simulink model "Tecs"  (R2023b)
settings: Solver=ode4  StartTime=0.0  StopTime=50  FixedStep=.02  RelTol=1e-3
values from neighbouring files (symbols this model uses):
  gravity = Airplane_data(52)    [Data_edit.m]
libraries: simulink x11
settings Model: Creator=Saif Mohamed  LastModifiedBy=saifg

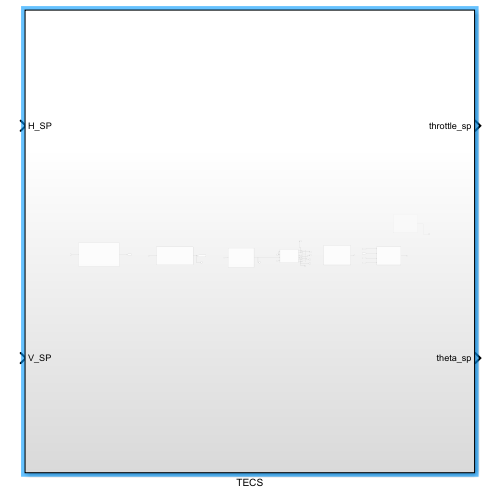
[thumbnail: Simulink's stored preview of the top-level diagram]
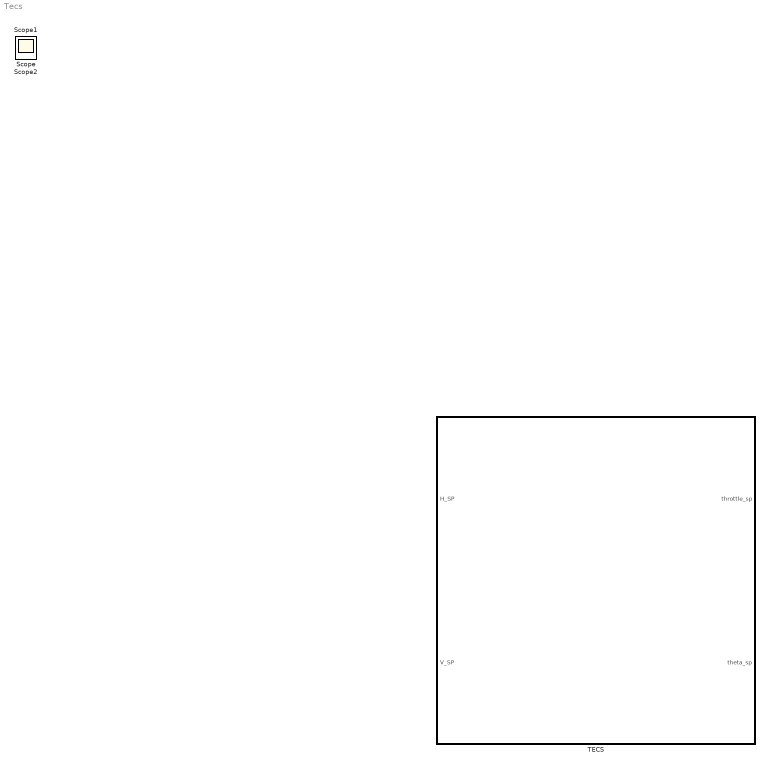
== system Tecs ==
  TECS : Subsystem
  Scope : Scope
  Scope1 : Scope
  Scope2 : Scope

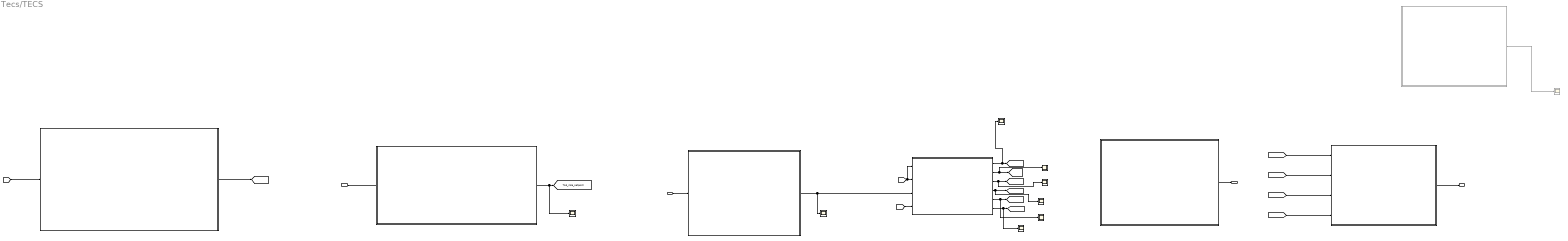
== system Tecs/TECS ==
  H_SP : Inport
  V_SP : Inport  Port=2
  Scope{,1..7} (8 alike) : Scope
  Scope9 : Scope  Commented=on
  _update_pitch_setpoint : Subsystem
  runAltitudeControllerSmoothVelocity : Subsystem
  update_energy_estimates : Subsystem
  update_pitch_setpoint : Subsystem  Commented=on
  update_speed_setpoint : Subsystem
  update_speed_states : Subsystem
  update_throttle_setpoint : Subsystem
  throttle_sp : Outport
  theta_sp : Outport  Port=2
  tag scope: SEB_error=global, SKE_rate=global, SKE_rate_setpoint=global, SPE_rate=global, SPE_rate_setpoint=global, STE_error=global, TAS_rate_setpoint=global, tas_state_output=global
  wires:
  update_speed_setpoint/1(TAS_rate_setpoint) -> Scope/1, [TAS_rate_setpoint]
  update_energy_estimates/4(SKE_rate_setpoint) -> Scope5/1, [SKE_rate_setpoint]
  update_energy_estimates/3(SPE_rate_setpoint) -> Scope4/1, [SPE_rate_setpoint]
  update_energy_estimates/5(SPE_rate) -> Scope6/1, [SPE_rate]
  update_speed_states/1(tas_state) -> [tas_state_output]  "tas_state"
  update_energy_estimates/6(SKE_rate) -> Scope7/1, [SKE_rate]
  V_SP/1 -> update_speed_setpoint/1(TAS_setpoint)
  update_energy_estimates/1(STE_error) -> Scope2/1, [STE_error]
  update_energy_estimates/2(SEB_error) -> Scope3/1, [SEB_error]
  update_pitch_setpoint/1(_last_pitch_setpoint) -> Scope9/1
  [Z] -> update_energy_estimates/1(hgt_setpoint), update_energy_estimates/2(vert_pos_state z from (6DoF))
  [w_e] -> update_energy_estimates/4(vert_vel_state)
  H_SP/1 -> runAltitudeControllerSmoothVelocity/1(H_Desired)
  runAltitudeControllerSmoothVelocity/1(hgt_rate_setpoint) -> Scope1/1, update_energy_estimates/3(hgt_rate_setpoint)
  update_throttle_setpoint/1(last_throttle_setpoint) -> throttle_sp/1
  [SPE_rate] -> _update_pitch_setpoint/2(SPE_Rate)
  _update_pitch_setpoint/1(_last_pitch_setpoint) -> theta_sp/1
  [SKE_rate] -> _update_pitch_setpoint/3(SKE_Rate)
  [SPE_rate_setpoint] -> _update_pitch_setpoint/1(SPE_rate_setpoint)
  [SKE_rate_setpoint] -> _update_pitch_setpoint/4(SKE_rate_setpoint)
  [V_tot] -> update_speed_states/1(EAS)

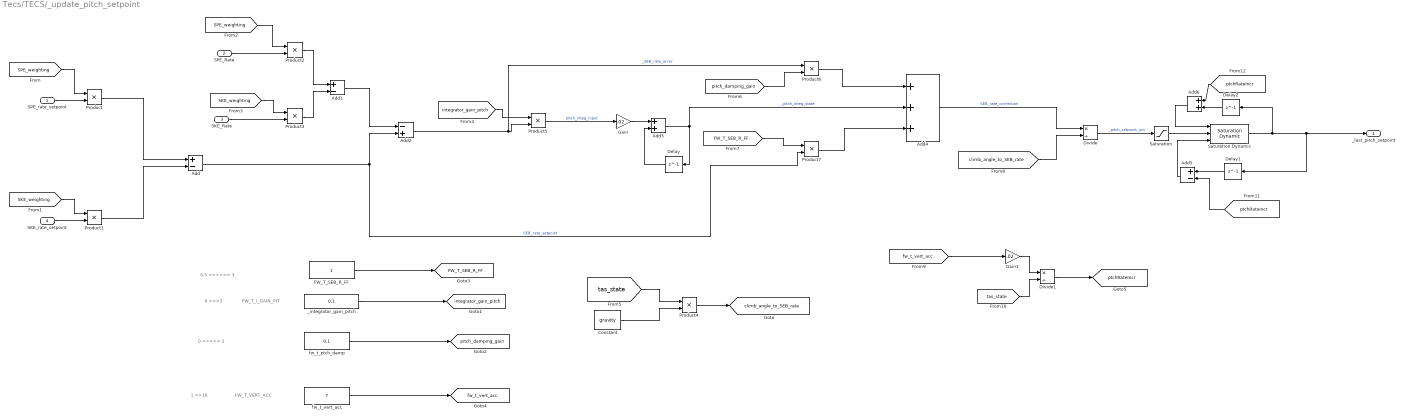
== system Tecs/TECS/_update_pitch_setpoint ==
  note: 0 >>>>> 2
  note: 0.5 >>>>>> 3
  note: FW_T_VERT_ACC
  note: 1 >>10
  note: 0 >>>2
  note: FW_T_I_GAIN_PIT
  SPE_rate_setpoint : Inport
  SPE_Rate : Inport  Port=2
  SKE_Rate : Inport  Port=3
  SKE_rate_setpoint : Inport  Port=4
  Add : Sum  Inputs=+-
  Add1 : Sum  Inputs=+-
  Add2 : Sum  Inputs=-+
  Add3 : Sum
  Add4 : Sum  Inputs=+++
  Add5 : Sum  Inputs=+-
  Add6 : Sum
  Constant : Constant  Value=gravity
  Delay : Delay  DelayLength=1
  Delay1 : Delay  DelayLength=1
  Delay2 : Delay  DelayLength=1
  Divide : Product  Inputs=*/
  Divide1 : Product  Inputs=*/
  FW_T_SEB_R_FF : Constant
  Gain : Gain  Gain=.02
  Gain1 : Gain  Gain=.02
  Product{,1..7} (8 alike) : Product
  Saturation : Saturate
  Saturation Dynamic : simulink/Discontinuities/Saturation Dynamic  OutMin=[]  OutMax=[]  OutDataTypeStr=Inherit: Same as second input  OutDataType=fixdt(1, 16)  OutScaling=2^-10  DoSatur=off
  _integrator_gain_pitch : Constant  Value=0.1
  fw_t_ptch_damp : Constant  Value=0.1
  fw_t_vert_acc : Constant  Value=7
  _last_pitch_setpoint : Outport
  tag scope: FW_T_SEB_R_FF=global, climb_angle_to_SEB_rate=global, fw_t_vert_acc=global, integrator_gain_pitch=global, pitch_damping_gain=global, ptchRateIncr=global
  wires:
  SKE_rate_setpoint/1 -> Product1/2
  SPE_rate_setpoint/1 -> Product/2
  Product/1 -> Add/1
  Product1/1 -> Add/2
  [SPE_weighting] -> Product/1
  [SKE_weighting] -> Product1/1
  SPE_Rate/1 -> Product2/2
  [SPE_weighting] -> Product2/1
  SKE_Rate/1 -> Product3/2
  [SKE_weighting] -> Product3/1
  Product3/1 -> Add1/2
  Product2/1 -> Add1/1
  Add/1 -> Product7/2, Add2/2  "SEB_rate_setpoint"
  Add1/1 -> Add2/1
  Add2/1 -> Product6/1, Product5/2  "_SEB_rate_error"
  [tas_state] -> Product4/1
  Constant/1 -> Product4/2
  Product4/1 -> [climb_angle_to_SEB_rate]
  _integrator_gain_pitch/1 -> [integrator_gain_pitch]
  [integrator_gain_pitch] -> Product5/1
  Product5/1 -> Gain/1  "pitch_integ_input"
  Gain/1 -> Add3/1
  Add3/1 -> Add4/2, Delay/1  "_pitch_integ_state"
  Delay/1 -> Add3/2
  fw_t_ptch_damp/1 -> [pitch_damping_gain]
  [pitch_damping_gain] -> Product6/2
  Product6/1 -> Add4/1
  FW_T_SEB_R_FF/1 -> [FW_T_SEB_R_FF]
  [FW_T_SEB_R_FF] -> Product7/1
  Product7/1 -> Add4/3
  Add4/1 -> Divide/1  "SEB_rate_correction"
  [climb_angle_to_SEB_rate] -> Divide/2
  Divide/1 -> Saturation/1  "_pitch_setpoint_unc"
  fw_t_vert_acc/1 -> [fw_t_vert_acc]
  [tas_state] -> Divide1/2
  [fw_t_vert_acc] -> Gain1/1
  Gain1/1 -> Divide1/1
  Divide1/1 -> [ptchRateIncr]
  Saturation/1 -> Saturation Dynamic/2
  Saturation Dynamic/1 -> Delay2/1, _last_pitch_setpoint/1, Delay1/1
  Delay1/1 -> Add5/1
  [ptchRateIncr] -> Add5/2
  Add5/1 -> Saturation Dynamic/3
  Delay2/1 -> Add6/2
  [ptchRateIncr] -> Add6/1
  Add6/1 -> Saturation Dynamic/1

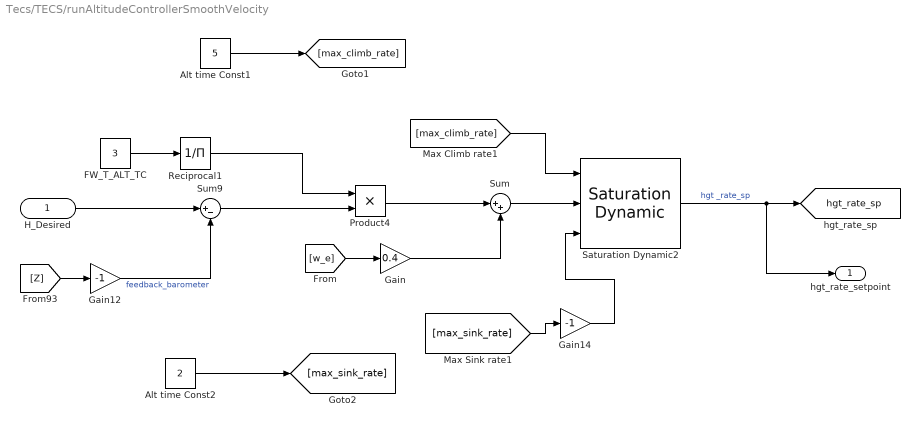
== system Tecs/TECS/runAltitudeControllerSmoothVelocity ==
  H_Desired : Inport
  Alt time Const1 : Constant  Value=5
  Alt time Const2 : Constant  Value=2
  FW_T_ALT_TC : Constant  Value=3
  Gain : Gain  Gain=0.4
  Gain12 : Gain  Gain=-1
  Gain14 : Gain  Gain=-1
  Product4 : Product
  Reciprocal1 : Product  Inputs=/
  Saturation Dynamic2 : simulink/Discontinuities/Saturation Dynamic  OutMin=[]  OutMax=[]  OutDataTypeStr=Inherit: Same as second input  OutDataType=fixdt(1, 16)  OutScaling=2^-10  DoSatur=off
  Sum : Sum  Inputs=|++
  Sum9 : Sum  Inputs=|+-
  hgt_rate_setpoint : Outport
  tag scope: hgt_rate_sp=global
  wires:
  Gain12/1 -> Sum9/2  "feedback_barometer"
  FW_T_ALT_TC/1 -> Reciprocal1/1
  H_Desired/1 -> Sum9/1
  [Z] -> Gain12/1
  Sum9/1 -> Product4/2
  [max_sink_rate] -> Gain14/1
  Reciprocal1/1 -> Product4/1
  Gain14/1 -> Saturation Dynamic2/3
  Saturation Dynamic2/1 -> hgt_rate_setpoint/1, [hgt_rate_sp]  "hgt _rate_sp"
  [max_climb_rate] -> Saturation Dynamic2/1
  Alt time Const1/1 -> [max_climb_rate]
  Alt time Const2/1 -> [max_sink_rate]
  [w_e] -> Gain/1
  Sum/1 -> Saturation Dynamic2/2
  Product4/1 -> Sum/1
  Gain/1 -> Sum/2

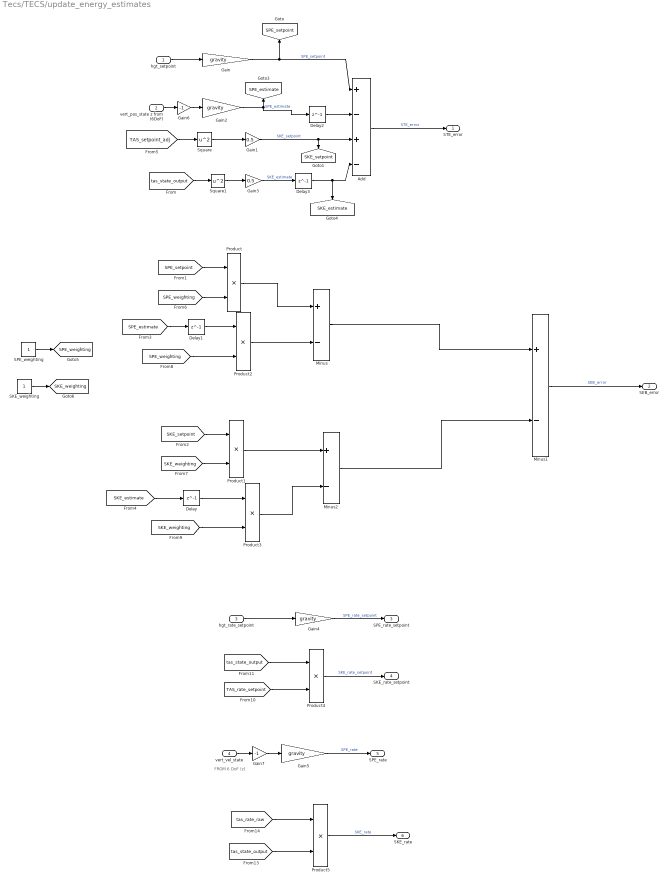
== system Tecs/TECS/update_energy_estimates ==
  note: FROM 6 DoF (z)
  hgt_setpoint : Inport
  vert_pos_state z from (6DoF) : Inport  Port=2
  hgt_rate_setpoint : Inport  Port=3
  vert_vel_state : Inport  Port=4
  Add : Sum  Inputs=+-+-
  Delay{,1..3} (4 alike) : Delay  DelayLength=1
  Gain{,2,4..5} (4 alike) : Gain  Gain=gravity
  Gain1 : Gain  Gain=0.5
  Gain3 : Gain  Gain=0.5
  Gain6 : Gain  Gain=-1
  Gain7 : Gain  Gain=-1
  Minus : Sum  Inputs=+-
  Minus1 : Sum  Inputs=+-
  Minus2 : Sum  Inputs=+-
  Product{,1..5} (6 alike) : Product
  SKE_weighting : Constant
  SPE_weighting : Constant
  Square : Math  Operator=square
  Square1 : Math  Operator=square
  STE_error : Outport
  SEB_error : Outport  Port=2
  SPE_rate_setpoint : Outport  Port=3
  SKE_rate_setpoint : Outport  Port=4
  SPE_rate : Outport  Port=5
  SKE_rate : Outport  Port=6
  tag scope: SKE_estimate=global, SKE_setpoint=global, SKE_weighting=global, SPE_estimate=global, SPE_setpoint=global, SPE_weighting=global
  wires:
  [SPE_weighting] -> Product2/2
  SKE_weighting/1 -> [SKE_weighting]
  [SKE_weighting] -> Product1/2
  vert_pos_state z from (6DoF)/1 -> Gain6/1
  [SKE_estimate] -> Delay/1
  [tas_rate_raw] -> Product5/1
  Square1/1 -> Gain3/1
  [SKE_setpoint] -> Product1/1
  [SPE_weighting] -> Product/2
  Product5/1 -> SKE_rate/1  "SKE_rate"
  [SKE_weighting] -> Product3/2
  [tas_state_output] -> Product4/1
  Gain3/1 -> Delay3/1  "SKE_estimate"
  hgt_setpoint/1 -> Gain/1
  Gain2/1 -> Delay2/1, [SPE_estimate]  "SPE_estimate"
  [tas_state_output] -> Square1/1
  [SPE_estimate] -> Delay1/1
  vert_vel_state/1 -> Gain7/1
  Minus/1 -> Minus1/1
  [tas_state_output] -> Product5/2
  Gain/1 -> Add/1, [SPE_setpoint]  "SPE_setpoint"
  Minus2/1 -> Minus1/2
  Gain1/1 -> [SKE_setpoint], Add/3  "SKE_setpoint"
  Product3/1 -> Minus2/2
  [TAS_setpoint_adj] -> Square/1
  Square/1 -> Gain1/1
  [SPE_setpoint] -> Product/1
  Product/1 -> Minus/1
  Add/1 -> STE_error/1  "STE_error"
  hgt_rate_setpoint/1 -> Gain4/1
  [TAS_rate_setpoint] -> Product4/2
  Gain5/1 -> SPE_rate/1  "SPE_rate"
  SPE_weighting/1 -> [SPE_weighting]
  Minus1/1 -> SEB_error/1  "SEB_error"
  Product4/1 -> SKE_rate_setpoint/1  "SKE_rate_setpoint"
  Gain4/1 -> SPE_rate_setpoint/1  "SPE_rate_setpoint"
  Delay/1 -> Product3/1
  Delay1/1 -> Product2/1
  Product2/1 -> Minus/2
  Product1/1 -> Minus2/1
  Gain6/1 -> Gain2/1
  Delay2/1 -> Add/2
  Delay3/1 -> Add/4, [SKE_estimate]
  Gain7/1 -> Gain5/1

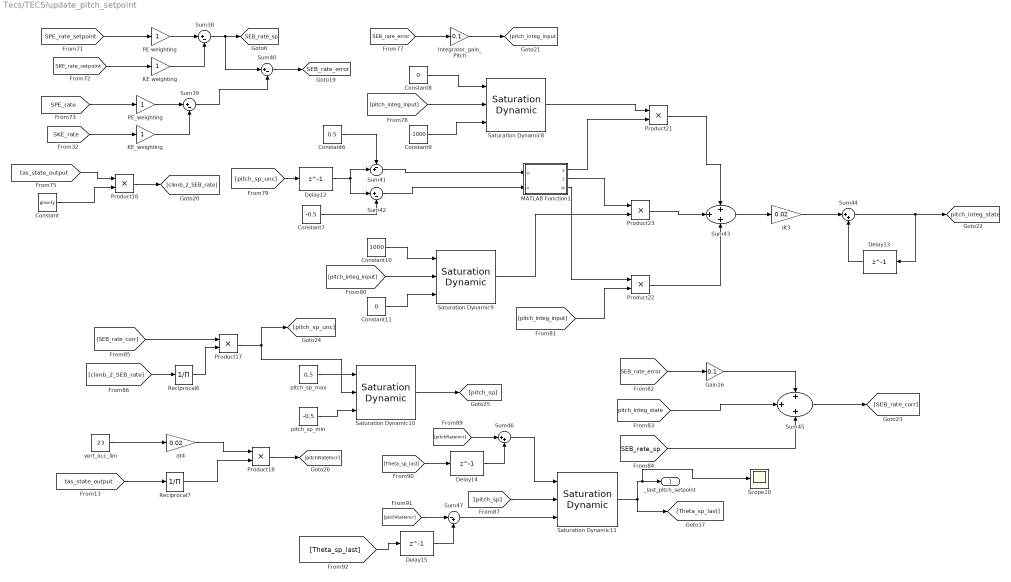
== system Tecs/TECS/update_pitch_setpoint ==
  Constant : Constant  Value=gravity
  Constant10 : Constant  Value=1000
  Constant11 : Constant  Value=0
  Constant6 : Constant  Value=0.5
  Constant7 : Constant  Value=-0.5
  Constant8 : Constant  Value=0
  Constant9 : Constant  Value=-1000
  Delay{12..15} (4 alike) : Delay  DelayLength=1  InitialCondition=0  UseCircularBuffer=on  SampleTime=0.02
  Gain16 : Gain  Gain=0.1
  Integrator_gain_Pitch : Gain  Gain=0.1
  KE weighting : Gain
  KE_weighting : Gain
  MATLAB Function1 : MATLAB Function  TreatAsAtomicUnit=on
  PE weighting : Gain
  PE_weighting : Gain
  Product{16..18,21..23} (6 alike) : Product
  Reciprocal6 : Product  Inputs=/
  Reciprocal7 : Product  Inputs=/
  Saturation Dynamic{8..11} (4 alike) : simulink/Discontinuities/Saturation Dynamic  OutMin=[]  OutMax=[]  OutDataTypeStr=Inherit: Same as second input  OutDataType=fixdt(1, 16)  OutScaling=2^-10  DoSatur=off
  Scope10 : Scope
  Sum{38..40,42} (4 alike) : Sum  Inputs=|+-
  Sum41 : Sum  Inputs=-+|
  Sum43 : Sum  Inputs=+++
  Sum44 : Sum  Inputs=|++
  Sum45 : Sum  Inputs=+++
  Sum46 : Sum  Inputs=|++
  Sum47 : Sum  Inputs=|-+
  dt3 : Gain  Gain=0.02
  dt4 : Gain  Gain=0.02
  pitch_sp_max : Constant  Value=0.5
  pitch_sp_min : Constant  Value=-0.5
  vert_acc_lim : Constant  Value=23
  _last_pitch_setpoint : Outport
  tag scope: SEB_rate_error=global, SEB_rate_sp=global, pitch_integ_state=global
  wires:
  Product18/1 -> [pitchRateIncr]
  Saturation Dynamic9/1 -> Product23/2
  [tas_state_output] -> Reciprocal7/1
  pitch_sp_min/1 -> Saturation Dynamic10/3
  [climb_2_SEB_rate] -> Reciprocal6/1
  KE weighting/1 -> Sum38/2
  Gain16/1 -> Sum45/1
  [SEB_rate_corr] -> Product17/1
  Reciprocal7/1 -> Product18/2
  pitch_sp_max/1 -> Saturation Dynamic10/1
  [pitch_integ_input] -> Product22/2
  [SPE_rate_setpoint] -> PE weighting/1
  PE weighting/1 -> Sum38/1
  Product16/1 -> [climb_2_SEB_rate]
  Reciprocal6/1 -> Product17/2
  Delay15/1 -> Sum47/2
  [pitchRateIncr] -> Sum47/1
  Sum46/1 -> Saturation Dynamic11/1
  Delay12/1 -> Sum42/1, Sum41/2
  Delay13/1 -> Sum44/2
  [SEB_rate_sp] -> Sum45/3
  [tas_state_output] -> Product16/1
  [SEB_rate_error] -> Gain16/1
  KE_weighting/1 -> Sum39/2
  MATLAB Function1/2(z) -> Product23/1
  [pitch_integ_input] -> Saturation Dynamic9/2
  [Theta_sp_last] -> Delay15/1
  Sum45/1 -> [SEB_rate_corr]
  Product23/1 -> Sum43/2
  Constant8/1 -> Saturation Dynamic8/1
  Sum43/1 -> dt3/1
  [SKE_rate_setpoint] -> KE weighting/1
  MATLAB Function1/3(w) -> Product22/1
  Sum40/1 -> [SEB_rate_error]
  vert_acc_lim/1 -> dt4/1
  Sum39/1 -> Sum40/2
  MATLAB Function1/1(y) -> Product21/2
  Constant10/1 -> Saturation Dynamic9/1
  [pitch_sp_unc] -> Delay12/1
  Saturation Dynamic11/1 -> _last_pitch_setpoint/1, Scope10/1, [Theta_sp_last]
  Constant11/1 -> Saturation Dynamic9/3
  dt3/1 -> Sum44/1
  [pitchRateIncr] -> Sum46/1
  Product22/1 -> Sum43/3
  [pitch_integ_state] -> Sum45/2
  Integrator_gain_Pitch/1 -> [pitch_integ_input]
  Constant6/1 -> Sum41/1
  Delay14/1 -> Sum46/2
  Saturation Dynamic8/1 -> Product21/1
  Constant9/1 -> Saturation Dynamic8/3
  Constant/1 -> Product16/2
  Product21/1 -> Sum43/1
  Sum44/1 -> Delay13/1, [pitch_integ_state]
  Sum42/1 -> MATLAB Function1/2(v)
  [SEB_rate_error] -> Integrator_gain_Pitch/1
  Product17/1 -> Saturation Dynamic10/2, [pitch_sp_unc]
  PE_weighting/1 -> Sum39/1
  Sum41/1 -> MATLAB Function1/1(u)
  [pitch_integ_input] -> Saturation Dynamic8/2
  Sum47/1 -> Saturation Dynamic11/3
  [pitch_sp] -> Saturation Dynamic11/2
  Sum38/1 -> Sum40/1, [SEB_rate_sp]
  Constant7/1 -> Sum42/2
  [SPE_rate] -> PE_weighting/1
  [SKE_rate] -> KE_weighting/1
  Saturation Dynamic10/1 -> [pitch_sp]
  dt4/1 -> Product18/1
  [Theta_sp_last] -> Delay14/1

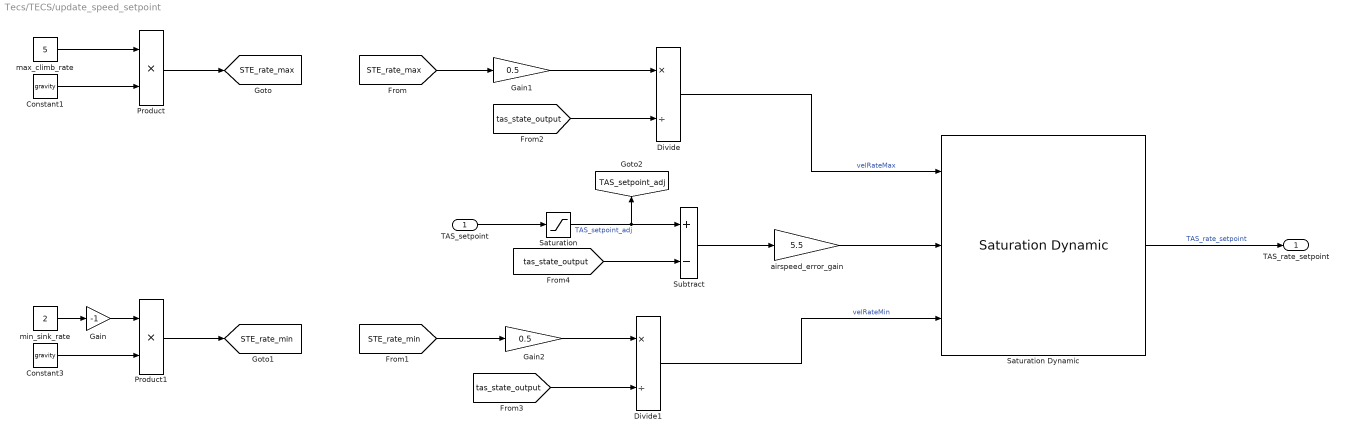
== system Tecs/TECS/update_speed_setpoint ==
  TAS_setpoint : Inport
  Constant1 : Constant  Value=gravity
  Constant3 : Constant  Value=gravity
  Divide : Product  Inputs=*/
  Divide1 : Product  Inputs=*/
  Gain : Gain  Gain=-1
  Gain1 : Gain  Gain=0.5
  Gain2 : Gain  Gain=0.5
  Product : Product
  Product1 : Product
  Saturation : Saturate  UpperLimit=50  LowerLimit=8
  Saturation Dynamic : simulink/Discontinuities/Saturation Dynamic  OutMin=[]  OutMax=[]  OutDataTypeStr=Inherit: Same as second input  OutDataType=fixdt(1, 16)  OutScaling=2^-10  DoSatur=off
  Subtract : Sum  Inputs=+-
  airspeed_error_gain : Gain  Gain=5.5
  max_climb_rate : Constant  Value=5
  min_sink_rate : Constant  Value=2
  TAS_rate_setpoint : Outport
  tag scope: STE_rate_max=global, STE_rate_min=global, TAS_setpoint_adj=global
  wires:
  Saturation Dynamic/1 -> TAS_rate_setpoint/1  "TAS_rate_setpoint"
  Divide1/1 -> Saturation Dynamic/3  "velRateMin"
  Gain2/1 -> Divide1/1
  Product/1 -> [STE_rate_max]
  [STE_rate_min] -> Gain2/1
  [tas_state_output] -> Divide1/2
  [STE_rate_max] -> Gain1/1
  airspeed_error_gain/1 -> Saturation Dynamic/2
  Divide/1 -> Saturation Dynamic/1  "velRateMax"
  Gain1/1 -> Divide/1
  [tas_state_output] -> Subtract/2
  Constant3/1 -> Product1/2
  max_climb_rate/1 -> Product/1
  min_sink_rate/1 -> Gain/1
  Saturation/1 -> Subtract/1, [TAS_setpoint_adj]  "TAS_setpoint_adj"
  Constant1/1 -> Product/2
  [tas_state_output] -> Divide/2
  TAS_setpoint/1 -> Saturation/1
  Subtract/1 -> airspeed_error_gain/1
  Product1/1 -> [STE_rate_min]
  Gain/1 -> Product1/1

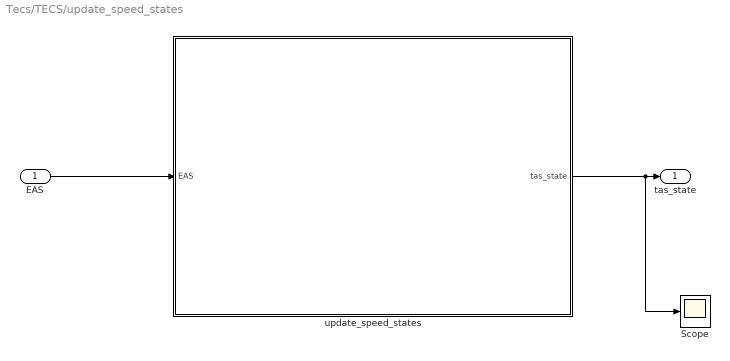
== system Tecs/TECS/update_speed_states ==
  EAS : Inport
  Scope : Scope
  update_speed_states : Subsystem
  tas_state : Outport
  wires:
  EAS/1 -> update_speed_states/1(EAS)
  update_speed_states/1(tas_state) -> Scope/1, tas_state/1

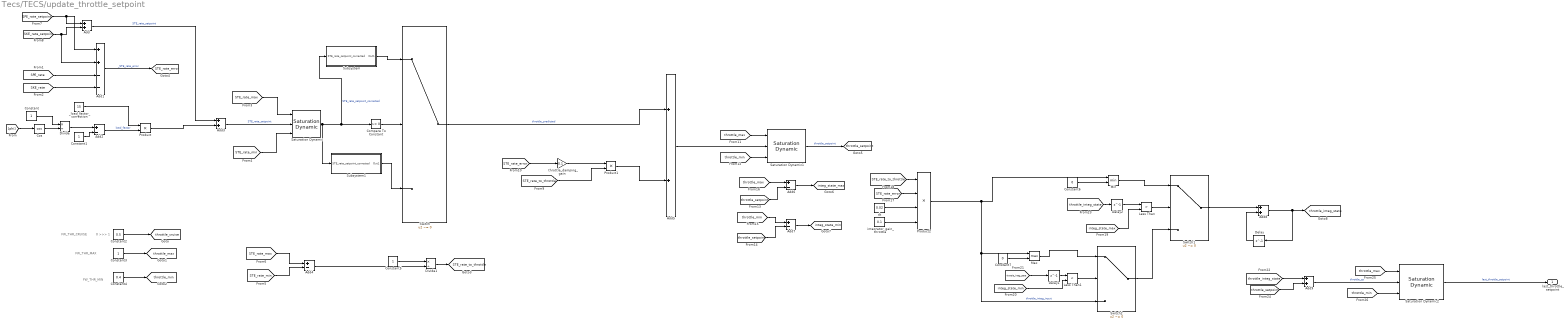
== system Tecs/TECS/update_throttle_setpoint ==
  note: FW_THR_MIN
  note: FW_THR_MAX
  note: FW_THR_CRUISE
  note: 0 >>> 1
  Add{,3,5,8..9} (5 alike) : Sum
  Add1 : Sum  Inputs=++--
  Add{2,4,6..7} (4 alike) : Sum  Inputs=+-
  Compare To Constant : simulink/Logic and Bit Operations/Compare To Constant  relop=>=  const=0  OutDataTypeStr=boolean
  Constant{,1,3,5} (4 alike) : Constant
  Constant2 : Constant  Value=0.5
  Constant4 : Constant  Value=0.4
  Constant6 : Constant  Value=0
  Constant7 : Constant  Value=0
  Cos : Trigonometry  Operator=cos
  Delay : Delay  DelayLength=1
  Delay1 : Delay  DelayLength=1
  Delay2 : Delay  DelayLength=1
  Divide : Product  Inputs=*/
  Divide1 : Product  Inputs=*/
  Less Than : RelationalOperator  Operator=>  OutDataTypeStr=boolean  RndMeth=Simplest  InputSameDT=off
  Less Than1 : RelationalOperator  Operator=<  OutDataTypeStr=boolean  RndMeth=Simplest  InputSameDT=off
  Max : MinMax  Function=max  Inputs=2
  Min : MinMax  Inputs=2
  Product : Product
  Product1 : Product
  Product2 : Product  Inputs=4
  Saturation Dynamic : simulink/Discontinuities/Saturation Dynamic  OutMin=[]  OutMax=[]  OutDataTypeStr=Inherit: Same as second input  OutDataType=fixdt(1, 16)  OutScaling=2^-10  DoSatur=off
  Saturation Dynamic1 : simulink/Discontinuities/Saturation Dynamic  OutMin=[]  OutMax=[]  OutDataTypeStr=Inherit: Same as second input  OutDataType=fixdt(1, 16)  OutScaling=2^-10  DoSatur=off
  Saturation Dynamic2 : simulink/Discontinuities/Saturation Dynamic  OutMin=[]  OutMax=[]  OutDataTypeStr=Inherit: Same as second input  OutDataType=fixdt(1, 16)  OutScaling=2^-10  DoSatur=off
  Subsystem : Subsystem
  Subsystem1 : Subsystem
  Switch : Switch  Criteria=u2 ~= 0  SaturateOnIntegerOverflow=off  InputSameDT=off
  Switch1 : Switch  Criteria=u2 ~= 0  SaturateOnIntegerOverflow=off  InputSameDT=off
  Switch2 : Switch  Criteria=u2 ~= 0  SaturateOnIntegerOverflow=off  InputSameDT=off
  _load_factor_correction : Constant  Value=15
  dt : Constant  Value=0.02
  integrator_gain_throttle : Constant  Value=0.1
  throttle_damping_gain : Gain  Gain=0.1
  last_throttle_setpoint : Outport
  tag scope: STE_rate_error=global, STE_rate_to_throttle=global, integ_state_max=global, integ_state_min=global, throttle_cruise=global, throttle_integ_state=global, throttle_max=global, throttle_min=global, throttle_setpoint=global
  wires:
  [SKE_rate_setpoint] -> Add1/2, Add/2
  [SPE_rate_setpoint] -> Add1/1, Add/1
  Add/1 -> Add3/1  "STE_rate_setpoint"
  [SPE_rate] -> Add1/3
  [SKE_rate] -> Add1/4
  Add1/1 -> [STE_rate_error]  "_STE_rate_error"
  [phi] -> Cos/1
  Cos/1 -> Divide/2
  Constant/1 -> Divide/1
  Divide/1 -> Add2/1
  Constant1/1 -> Add2/2
  Add2/1 -> Product/2  "load_factor"
  _load_factor_correction/1 -> Product/1
  Product/1 -> Add3/2
  Add3/1 -> Saturation Dynamic/2  "STE_rate_setpoint"
  [STE_rate_max] -> Saturation Dynamic/1
  [STE_rate_min] -> Saturation Dynamic/3
  Saturation Dynamic/1 -> Subsystem1/1(STE_rate_setpoint_corrected), Subsystem/1(STE_rate_setpoint_corrected), Compare To Constant/1  "STE_rate_setpoint_corrected"
  Compare To Constant/1 -> Switch/2
  Constant4/1 -> [throttle_min]
  Constant3/1 -> [throttle_max]
  Constant2/1 -> [throttle_cruise]
  Subsystem/1(Out1) -> Switch/1
  Subsystem1/1(Out1) -> Switch/3
  Switch/1 -> Add5/1  "throttle_predicted"
  [STE_rate_max] -> Add4/1
  [STE_rate_min] -> Add4/2
  Add4/1 -> Divide1/2
  Constant5/1 -> Divide1/1
  Divide1/1 -> [STE_rate_to_throttle]
  [STE_rate_error] -> throttle_damping_gain/1
  throttle_damping_gain/1 -> Product1/1
  [STE_rate_to_throttle] -> Product1/2
  Product1/1 -> Add5/2
  Add5/1 -> Saturation Dynamic1/2
  [throttle_max] -> Saturation Dynamic1/1
  [throttle_min] -> Saturation Dynamic1/3
  Saturation Dynamic1/1 -> [throttle_setpoint]  "throttle_setpoint"
  [throttle_max] -> Add6/1
  [throttle_setpoint] -> Add6/2
  Add6/1 -> [integ_state_max]
  [throttle_min] -> Add7/1
  [throttle_setpoint] -> Add7/2
  Add7/1 -> [integ_state_min]
  integrator_gain_throttle/1 -> Product2/4
  dt/1 -> Product2/3
  [STE_rate_error] -> Product2/2
  [STE_rate_to_throttle] -> Product2/1
  Product2/1 -> Min/1, Max/1, Switch2/3  "throttle_integ_input"
  [integ_state_max] -> Less Than/2
  Less Than/1 -> Switch1/2
  Constant6/1 -> Min/2
  Min/1 -> Switch1/1
  Switch2/1 -> Switch1/3
  Less Than1/1 -> Switch2/2
  [integ_state_min] -> Less Than1/2
  Max/1 -> Switch2/1
  Constant7/1 -> Max/2
  Switch1/1 -> Add8/1
  Add8/1 -> [throttle_integ_state], Delay/1
  Delay/1 -> Add8/2
  [throttle_integ_state] -> Delay2/1
  [throttle_integ_state] -> Delay1/1
  [throttle_setpoint] -> Add9/2
  [throttle_integ_state] -> Add9/1
  Add9/1 -> Saturation Dynamic2/2  "throttle_sp"
  [throttle_min] -> Saturation Dynamic2/3
  [throttle_max] -> Saturation Dynamic2/1
  Saturation Dynamic2/1 -> last_throttle_setpoint/1  "last_throttle_setpoint"
  Delay1/1 -> Less Than1/1
  Delay2/1 -> Less Than/1

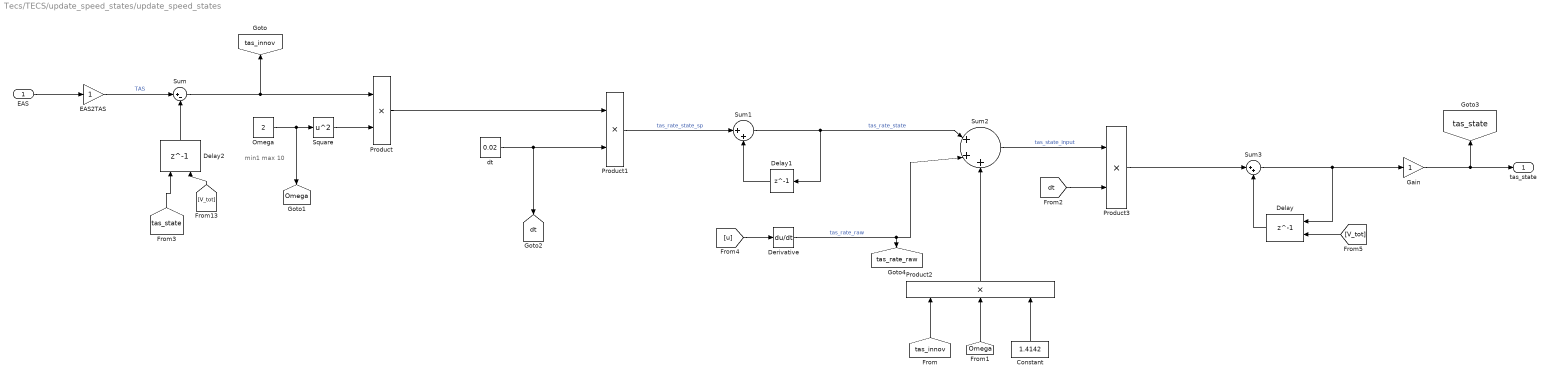
== system Tecs/TECS/update_speed_states/update_speed_states ==
  note: min1 max 10
  EAS : Inport
  Constant : Constant  Value=1.4142
  Delay : Delay  DelayLength=1  InitialConditionSource=Input port
      settings: InputPortMap=u0,p4
  Delay1 : Delay  DelayLength=1
  Delay2 : Delay  DelayLength=1  InitialConditionSource=Input port
      settings: InputPortMap=u0,p4
  Derivative : Derivative
  EAS2TAS : Gain
  Gain : Gain
  Omega : Constant  Value=2
  Product : Product
  Product1 : Product
  Product2 : Product  Inputs=3
  Product3 : Product
  Square : Math  Operator=square
  Sum : Sum  Inputs=|+-
  Sum1 : Sum  Inputs=|++
  Sum2 : Sum  Inputs=|+++
  Sum3 : Sum  Inputs=|++
  dt : Constant  Value=0.02
  tas_state : Outport
  tag scope: Omega=global, dt=global, tas_innov=global, tas_rate_raw=global, tas_state=global
  wires:
  Product1/1 -> Sum1/1  "tas_rate_state_sp"
  Sum1/1 -> Delay1/1, Sum2/1  "tas_rate_state"
  [tas_innov] -> Product2/1
  [dt] -> Product3/2
  Product2/1 -> Sum2/3
  Omega/1 -> Square/1, [Omega]
  dt/1 -> [dt], Product1/2
  [tas_state] -> Delay2/1
  Delay1/1 -> Sum1/2
  Sum2/1 -> Product3/1  "tas_state_input"
  [Omega] -> Product2/2
  Constant/1 -> Product2/3
  Square/1 -> Product/2
  Product/1 -> Product1/1
  [u] -> Derivative/1
  Derivative/1 -> Sum2/2, [tas_rate_raw]  "tas_rate_raw"
  [V_tot] -> Delay2/2
  [V_tot] -> Delay/2
  EAS/1 -> EAS2TAS/1
  Gain/1 -> tas_state/1, [tas_state]
  Product3/1 -> Sum3/1
  Delay/1 -> Sum3/2
  Sum3/1 -> Delay/1, Gain/1
  Delay2/1 -> Sum/2
  EAS2TAS/1 -> Sum/1  "TAS"
  Sum/1 -> Product/1, [tas_innov]

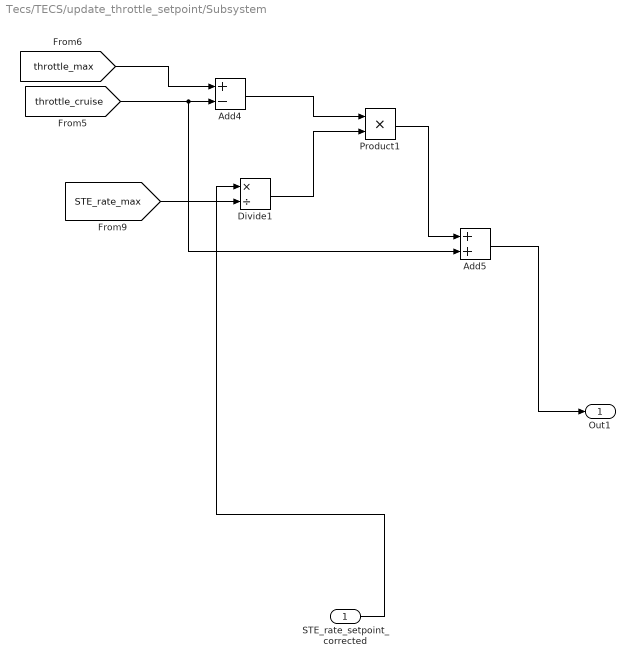
== system Tecs/TECS/update_throttle_setpoint/Subsystem ==
  STE_rate_setpoint_corrected : Inport
  Add4 : Sum  Inputs=+-
  Add5 : Sum
  Divide1 : Product  Inputs=*/
  Product1 : Product
  Out1 : Outport
  wires:
  [throttle_cruise] -> Add5/2, Add4/2
  Product1/1 -> Add5/1
  [STE_rate_max] -> Divide1/2
  [throttle_max] -> Add4/1
  Add4/1 -> Product1/1
  Divide1/1 -> Product1/2
  Add5/1 -> Out1/1
  STE_rate_setpoint_corrected/1 -> Divide1/1

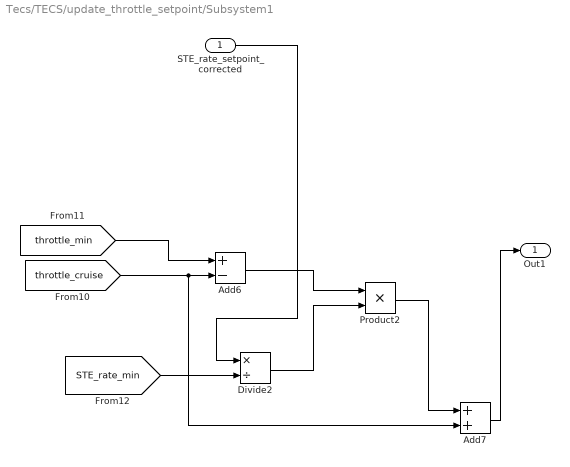
== system Tecs/TECS/update_throttle_setpoint/Subsystem1 ==
  STE_rate_setpoint_corrected : Inport
  Add6 : Sum  Inputs=+-
  Add7 : Sum
  Divide2 : Product  Inputs=*/
  Product2 : Product
  Out1 : Outport
  wires:
  Add7/1 -> Out1/1
  [throttle_min] -> Add6/1
  [STE_rate_min] -> Divide2/2
  STE_rate_setpoint_corrected/1 -> Divide2/1
  Add6/1 -> Product2/1
  [throttle_cruise] -> Add6/2, Add7/2
  Product2/1 -> Add7/1
  Divide2/1 -> Product2/2

== matlab function Tecs/TECS/update_pitch_setpoint/MATLAB Function1 ==
  data: u input; y output; z output; v input; w output
function [y,z,w] = fcn(u,v)
if u>0
    y=1;
    z=0;
    w=0;
elseif v<0
    y=0;
    z=1;
    w=0;
else 
    y=0;
    z=0;
    w=1;
end
